simulink model "Coupled_Model_crosslinked_intext"  (R2016a)
settings: Solver=FixedStepDiscrete  StartTime=0  StopTime=1000  FixedStep=1  RelTol=1e-3
undefined symbols (not defined in the file or in its folder): DiscIntNeverNeededParam
libraries: simulink_extras x32
(part 3 of 3)

== matlab function Coupled_Model_crosslinked_intext/kMtcontrol/kMtcontrol2/Spring Function ==
  data: popped output; Lspr input; F output; thresh input; K1 input
function [popped, F] = fcn(Lspr,thresh,K1)
%#eml

rest=0.2e-6;
popLength=0.45e-6;
springLength=0.8e-6;


K2=K1*springLength/(springLength+popLength);

popped=false;


if Lspr < thresh
    F=K1*(Lspr-rest);
    popped=false;

elseif Lspr >= thresh
    F=K2*(Lspr-rest-popLength);
    popped=true;
    
else
    F=0;
end

end

== matlab function Coupled_Model_crosslinked_intext/kMtcontrol/kMtcontrol2/Spring Function  ==
  data: popped output; Lspr input; F output; thresh input; K1 input
function [popped, F] = fcn(Lspr,thresh,K1)
%#eml

rest=0.2e-6;
popLength=0.45e-6;
springLength=0.8e-6;


K2=K1*springLength/(springLength+popLength);

popped=false;


if Lspr < thresh
    F=K1*(Lspr-rest);
    popped=false;

elseif Lspr >= thresh
    F=K2*(Lspr-rest-popLength);
    popped=true;
    
else
    F=0;
end

end

== matlab function Coupled_Model_crosslinked_intext/kMtcontrol/kMtcontrol2/kMt  Dynamics/kMtState/Left Catastophe Function ==
  data: u input; y output
function y = fcn(u)
%#eml
if u < 8e-7
y = -.65*((u*10^6)-0.75).^2+(23/60);
else 
    y=0.389;
end
y=abs(y);

== matlab function Coupled_Model_crosslinked_intext/kMtcontrol/kMtcontrol2/kMt  Dynamics/kMtState/Left Rescue Function ==
  data: u input; y output; v input
function y = fcn(u,v)
%#eml
if v<=0.05e-6
    y=1;
else
    y=-9.5e9*(u)+0.21;
end
y=abs(y);

== matlab function Coupled_Model_crosslinked_intext/kMtcontrol/kMtcontrol2/kMt  Dynamics/kMtState/Right Catastophe Function ==
  data: u input; y output
function y = fcn(u)
%#eml
if u < 8e-7
y = -.65*((u*10^6)-0.75).^2+(23/60);
else 
    y=.389;
end
y=abs(y);

== matlab function Coupled_Model_crosslinked_intext/kMtcontrol/kMtcontrol2/kMt  Dynamics/kMtState/Right Rescue Function ==
  data: u input; y output; v input
function y = fcn(u,v)
%#eml
if v<=0.05e-6
    y=1;
else
    y=-9.5e9*(u)+0.21;
end
y=abs(y);

== matlab function Coupled_Model_crosslinked_intext/kMtcontrol/kMtcontrol2/kMt Dynamics/kMtState/Left Catastophe Function ==
  data: u input; y output
function y = fcn(u)
%#eml
if u < 8e-7
y = -.65*((u*10^6)-0.75).^2+(23/60);
else 
    y=0.389;
end
y=abs(y);

== matlab function Coupled_Model_crosslinked_intext/kMtcontrol/kMtcontrol2/kMt Dynamics/kMtState/Left Rescue Function ==
  data: u input; y output; v input
function y = fcn(u,v)
%#eml
if v<=0.05e-6
    y=1;
else
    y=-9.5e9*(u)+0.21;
end
y=abs(y);

== matlab function Coupled_Model_crosslinked_intext/kMtcontrol/kMtcontrol2/kMt Dynamics/kMtState/Right Catastophe Function ==
  data: u input; y output
function y = fcn(u)
%#eml
if u < 8e-7
y = -.65*((u*10^6)-0.75).^2+(23/60);
else 
    y=.389;
end
y=abs(y);

== matlab function Coupled_Model_crosslinked_intext/kMtcontrol/kMtcontrol2/kMt Dynamics/kMtState/Right Rescue Function ==
  data: u input; y output; v input
function y = fcn(u,v)
%#eml
if v<=0.05e-6
    y=1;
else
    y=-9.5e9*(u)+0.21;
end
y=abs(y);

== matlab function Coupled_Model_crosslinked_intext/kMtcontrol/kMtcontrol2/kMt Dynamics /kMtState/Left Catastophe Function ==
  data: u input; y output
function y = fcn(u)
%#eml
if u < 8e-7
y = -.65*((u*10^6)-0.75).^2+(23/60);
else 
    y=0.389;
end
y=abs(y);

== matlab function Coupled_Model_crosslinked_intext/kMtcontrol/kMtcontrol2/kMt Dynamics /kMtState/Left Rescue Function ==
  data: u input; y output; v input
function y = fcn(u,v)
%#eml
if v<=0.05e-6
    y=1;
else
    y=-9.5e9*(u)+0.21;
end
y=abs(y);

== matlab function Coupled_Model_crosslinked_intext/kMtcontrol/kMtcontrol2/kMt Dynamics /kMtState/Right Catastophe Function ==
  data: u input; y output
function y = fcn(u)
%#eml
if u < 8e-7
y = -.65*((u*10^6)-0.75).^2+(23/60);
else 
    y=.389;
end
y=abs(y);

== matlab function Coupled_Model_crosslinked_intext/kMtcontrol/kMtcontrol2/kMt Dynamics /kMtState/Right Rescue Function ==
  data: u input; y output; v input
function y = fcn(u,v)
%#eml
if v<=0.05e-6
    y=1;
else
    y=-9.5e9*(u)+0.21;
end
y=abs(y);

== matlab function Coupled_Model_crosslinked_intext/kMtcontrol/kMtcontrol2/kMt Dynamics  /kMtState/Left Catastophe Function ==
  data: u input; y output
function y = fcn(u)
%#eml
if u < 8e-7
y = -.65*((u*10^6)-0.75).^2+(23/60);
else 
    y=0.389;
end
y=abs(y);

== matlab function Coupled_Model_crosslinked_intext/kMtcontrol/kMtcontrol2/kMt Dynamics  /kMtState/Left Rescue Function ==
  data: u input; y output; v input
function y = fcn(u,v)
%#eml
if v<=0.05e-6
    y=1;
else
    y=-9.5e9*(u)+0.21;
end
y=abs(y);

== matlab function Coupled_Model_crosslinked_intext/kMtcontrol/kMtcontrol2/kMt Dynamics  /kMtState/Right Catastophe Function ==
  data: u input; y output
function y = fcn(u)
%#eml
if u < 8e-7
y = -.65*((u*10^6)-0.75).^2+(23/60);
else 
    y=.389;
end
y=abs(y);

== matlab function Coupled_Model_crosslinked_intext/kMtcontrol/kMtcontrol2/kMt Dynamics  /kMtState/Right Rescue Function ==
  data: u input; y output; v input
function y = fcn(u,v)
%#eml
if v<=0.05e-6
    y=1;
else
    y=-9.5e9*(u)+0.21;
end
y=abs(y);

== matlab function Coupled_Model_crosslinked_intext/kMtcontrol/kMtcontrol3/ Spring Function ==
  data: popped output; Lspr input; F output; thresh input; K1 input
function [popped, F] = fcn(Lspr,thresh,K1)
%#eml

rest=0.2e-6;
popLength=0.45e-6;
springLength=0.8e-6;


K2=K1*springLength/(springLength+popLength);

popped=false;


if Lspr < thresh
    F=K1*(Lspr-rest);
    popped=false;

elseif Lspr >= thresh
    F=K2*(Lspr-rest-popLength);
    popped=true;
    
else
    F=0;
end

end

== matlab function Coupled_Model_crosslinked_intext/kMtcontrol/kMtcontrol3/ Spring Function  ==
  data: popped output; Lspr input; F output; thresh input; K1 input
function [popped, F] = fcn(Lspr,thresh,K1)
%#eml

rest=0.2e-6;
popLength=0.45e-6;
springLength=0.8e-6;


K2=K1*springLength/(springLength+popLength);

popped=false;


if Lspr < thresh
    F=K1*(Lspr-rest);
    popped=false;

elseif Lspr >= thresh
    F=K2*(Lspr-rest-popLength);
    popped=true;
    
else
    F=0;
end

end

== matlab function Coupled_Model_crosslinked_intext/kMtcontrol/kMtcontrol3/Spring Function ==
  data: popped output; Lspr input; F output; thresh input; K1 input
function [popped, F] = fcn(Lspr,thresh,K1)
%#eml

rest=0.2e-6;
popLength=0.45e-6;
springLength=0.8e-6;


K2=K1*springLength/(springLength+popLength);

popped=false;


if Lspr < thresh
    F=K1*(Lspr-rest);
    popped=false;

elseif Lspr >= thresh
    F=K2*(Lspr-rest-popLength);
    popped=true;
    
else
    F=0;
end

end

== matlab function Coupled_Model_crosslinked_intext/kMtcontrol/kMtcontrol3/Spring Function  ==
  data: popped output; Lspr input; F output; thresh input; K1 input
function [popped, F] = fcn(Lspr,thresh,K1)
%#eml

rest=0.2e-6;
popLength=0.45e-6;
springLength=0.8e-6;


K2=K1*springLength/(springLength+popLength);

popped=false;


if Lspr < thresh
    F=K1*(Lspr-rest);
    popped=false;

elseif Lspr >= thresh
    F=K2*(Lspr-rest-popLength);
    popped=true;
    
else
    F=0;
end

end

== matlab function Coupled_Model_crosslinked_intext/kMtcontrol/kMtcontrol3/kMt  Dynamics/kMtState/Left Catastophe Function ==
  data: u input; y output
function y = fcn(u)
%#eml
if u < 8e-7
y = -.65*((u*10^6)-0.75).^2+(23/60);
else 
    y=0.389;
end
y=abs(y);

== matlab function Coupled_Model_crosslinked_intext/kMtcontrol/kMtcontrol3/kMt  Dynamics/kMtState/Left Rescue Function ==
  data: u input; y output; v input
function y = fcn(u,v)
%#eml
if v<=0.05e-6
    y=1;
else
    y=-9.5e9*(u)+0.21;
end
y=abs(y);

== matlab function Coupled_Model_crosslinked_intext/kMtcontrol/kMtcontrol3/kMt  Dynamics/kMtState/Right Catastophe Function ==
  data: u input; y output
function y = fcn(u)
%#eml
if u < 8e-7
y = -.65*((u*10^6)-0.75).^2+(23/60);
else 
    y=.389;
end
y=abs(y);

== matlab function Coupled_Model_crosslinked_intext/kMtcontrol/kMtcontrol3/kMt  Dynamics/kMtState/Right Rescue Function ==
  data: u input; y output; v input
function y = fcn(u,v)
%#eml
if v<=0.05e-6
    y=1;
else
    y=-9.5e9*(u)+0.21;
end
y=abs(y);

== matlab function Coupled_Model_crosslinked_intext/kMtcontrol/kMtcontrol3/kMt Dynamics/kMtState/Left Catastophe Function ==
  data: u input; y output
function y = fcn(u)
%#eml
if u < 8e-7
y = -.65*((u*10^6)-0.75).^2+(23/60);
else 
    y=0.389;
end
y=abs(y);

== matlab function Coupled_Model_crosslinked_intext/kMtcontrol/kMtcontrol3/kMt Dynamics/kMtState/Left Rescue Function ==
  data: u input; y output; v input
function y = fcn(u,v)
%#eml
if v<=0.05e-6
    y=1;
else
    y=-9.5e9*(u)+0.21;
end
y=abs(y);

== matlab function Coupled_Model_crosslinked_intext/kMtcontrol/kMtcontrol3/kMt Dynamics/kMtState/Right Catastophe Function ==
  data: u input; y output
function y = fcn(u)
%#eml
if u < 8e-7
y = -.65*((u*10^6)-0.75).^2+(23/60);
else 
    y=.389;
end
y=abs(y);

== matlab function Coupled_Model_crosslinked_intext/kMtcontrol/kMtcontrol3/kMt Dynamics/kMtState/Right Rescue Function ==
  data: u input; y output; v input
function y = fcn(u,v)
%#eml
if v<=0.05e-6
    y=1;
else
    y=-9.5e9*(u)+0.21;
end
y=abs(y);

== matlab function Coupled_Model_crosslinked_intext/kMtcontrol/kMtcontrol3/kMt Dynamics /kMtState/Left Catastophe Function ==
  data: u input; y output
function y = fcn(u)
%#eml
if u < 8e-7
y = -.65*((u*10^6)-0.75).^2+(23/60);
else 
    y=0.389;
end
y=abs(y);

== matlab function Coupled_Model_crosslinked_intext/kMtcontrol/kMtcontrol3/kMt Dynamics /kMtState/Left Rescue Function ==
  data: u input; y output; v input
function y = fcn(u,v)
%#eml
if v<=0.05e-6
    y=1;
else
    y=-9.5e9*(u)+0.21;
end
y=abs(y);

== matlab function Coupled_Model_crosslinked_intext/kMtcontrol/kMtcontrol3/kMt Dynamics /kMtState/Right Catastophe Function ==
  data: u input; y output
function y = fcn(u)
%#eml
if u < 8e-7
y = -.65*((u*10^6)-0.75).^2+(23/60);
else 
    y=.389;
end
y=abs(y);

== matlab function Coupled_Model_crosslinked_intext/kMtcontrol/kMtcontrol3/kMt Dynamics /kMtState/Right Rescue Function ==
  data: u input; y output; v input
function y = fcn(u,v)
%#eml
if v<=0.05e-6
    y=1;
else
    y=-9.5e9*(u)+0.21;
end
y=abs(y);

== matlab function Coupled_Model_crosslinked_intext/kMtcontrol/kMtcontrol3/kMt Dynamics  /kMtState/Left Catastophe Function ==
  data: u input; y output
function y = fcn(u)
%#eml
if u < 8e-7
y = -.65*((u*10^6)-0.75).^2+(23/60);
else 
    y=0.389;
end
y=abs(y);

== matlab function Coupled_Model_crosslinked_intext/kMtcontrol/kMtcontrol3/kMt Dynamics  /kMtState/Left Rescue Function ==
  data: u input; y output; v input
function y = fcn(u,v)
%#eml
if v<=0.05e-6
    y=1;
else
    y=-9.5e9*(u)+0.21;
end
y=abs(y);

== matlab function Coupled_Model_crosslinked_intext/kMtcontrol/kMtcontrol3/kMt Dynamics  /kMtState/Right Catastophe Function ==
  data: u input; y output
function y = fcn(u)
%#eml
if u < 8e-7
y = -.65*((u*10^6)-0.75).^2+(23/60);
else 
    y=.389;
end
y=abs(y);

== matlab function Coupled_Model_crosslinked_intext/kMtcontrol/kMtcontrol3/kMt Dynamics  /kMtState/Right Rescue Function ==
  data: u input; y output; v input
function y = fcn(u,v)
%#eml
if v<=0.05e-6
    y=1;
else
    y=-9.5e9*(u)+0.21;
end
y=abs(y);

== matlab function Coupled_Model_crosslinked_intext/kMtcontrol/kMtcontrol/kMt Dynamics /kMtState/Left Catastophe Function ==
  data: u input; y output
function y = fcn(u)
%#eml
if u < 8e-7
y = -.65*((u*10^6)-0.75).^2+(23/60);
else 
    y=0.389;
end
y=abs(y);

== matlab function Coupled_Model_crosslinked_intext/kMtcontrol/kMtcontrol/kMt Dynamics /kMtState/Left Rescue Function ==
  data: u input; y output; v input
function y = fcn(u,v)
%#eml
if v<=0.05e-6
    y=1;
else
    y=-9.5e9*(u)+0.21;
end
y=abs(y);

== matlab function Coupled_Model_crosslinked_intext/kMtcontrol/kMtcontrol/kMt Dynamics /kMtState/Right Catastophe Function ==
  data: u input; y output
function y = fcn(u)
%#eml
if u < 8e-7
y = -.65*((u*10^6)-0.75).^2+(23/60);
else 
    y=.389;
end
y=abs(y);

== matlab function Coupled_Model_crosslinked_intext/kMtcontrol/kMtcontrol/kMt Dynamics /kMtState/Right Rescue Function ==
  data: u input; y output; v input
function y = fcn(u,v)
%#eml
if v<=0.05e-6
    y=1;
else
    y=-9.5e9*(u)+0.21;
end
y=abs(y);

== matlab function Coupled_Model_crosslinked_intext/kMtcontrol/kMtcontrol/kMt  Dynamics/kMtState/Left Catastophe Function ==
  data: u input; y output
function y = fcn(u)
%#eml
if u < 8e-7
y = -.65*((u*10^6)-0.75).^2+(23/60);
else 
    y=0.389;
end
y=abs(y);

== matlab function Coupled_Model_crosslinked_intext/kMtcontrol/kMtcontrol/kMt  Dynamics/kMtState/Left Rescue Function ==
  data: u input; y output; v input
function y = fcn(u,v)
%#eml
if v<=0.05e-6
    y=1;
else
    y=-9.5e9*(u)+0.21;
end
y=abs(y);

== matlab function Coupled_Model_crosslinked_intext/kMtcontrol/kMtcontrol/kMt  Dynamics/kMtState/Right Catastophe Function ==
  data: u input; y output
function y = fcn(u)
%#eml
if u < 8e-7
y = -.65*((u*10^6)-0.75).^2+(23/60);
else 
    y=.389;
end
y=abs(y);

== matlab function Coupled_Model_crosslinked_intext/kMtcontrol/kMtcontrol/kMt  Dynamics/kMtState/Right Rescue Function ==
  data: u input; y output; v input
function y = fcn(u,v)
%#eml
if v<=0.05e-6
    y=1;
else
    y=-9.5e9*(u)+0.21;
end
y=abs(y);

== matlab function Coupled_Model_crosslinked_intext/kMtcontrol/kMtcontrol/kMt Dynamics  /kMtState/Left Catastophe Function ==
  data: u input; y output
function y = fcn(u)
%#eml
if u < 8e-7
y = -.65*((u*10^6)-0.75).^2+(23/60);
else 
    y=0.389;
end
y=abs(y);

== matlab function Coupled_Model_crosslinked_intext/kMtcontrol/kMtcontrol/kMt Dynamics  /kMtState/Left Rescue Function ==
  data: u input; y output; v input
function y = fcn(u,v)
%#eml
if v<=0.05e-6
    y=1;
else
    y=-9.5e9*(u)+0.21;
end
y=abs(y);

== matlab function Coupled_Model_crosslinked_intext/kMtcontrol/kMtcontrol/kMt Dynamics  /kMtState/Right Catastophe Function ==
  data: u input; y output
function y = fcn(u)
%#eml
if u < 8e-7
y = -.65*((u*10^6)-0.75).^2+(23/60);
else 
    y=.389;
end
y=abs(y);

== matlab function Coupled_Model_crosslinked_intext/kMtcontrol/kMtcontrol/kMt Dynamics  /kMtState/Right Rescue Function ==
  data: u input; y output; v input
function y = fcn(u,v)
%#eml
if v<=0.05e-6
    y=1;
else
    y=-9.5e9*(u)+0.21;
end
y=abs(y);

== matlab function Coupled_Model_crosslinked_intext/Polcontrol/Embedded MATLAB Function2 ==
  data: Fnet input; Vip output
function Vip=fcn(Fnet)
%#eml

% if Fnet < 6e-12
    Vip=(50e-9/6e-12)*Fnet;
% else
%     Vip=50e-9;
% end

== matlab function Coupled_Model_crosslinked_intext/Polcontrol/Embedded MATLAB Function3 ==
  data: Fnet input; y output; Nmotors input
function y = fcn(Fnet,Nmotors)
%#eml
if Nmotors == 0
    y = 0;
else
    y = Fnet/Nmotors;
end

== matlab function Coupled_Model_crosslinked_intext/kMtcontrol/kMtcontrol/Spring Function ==
  data: popped output; Lspr input; F output; thresh input; K1 input
function [popped, F] = fcn(Lspr,thresh,K1)
%#eml

rest=0.2e-6;
popLength=0.45e-6;
springLength=0.8e-6;


K2=K1*springLength/(springLength+popLength);

popped=false;


if Lspr < thresh
    F=K1*(Lspr-rest);
    popped=false;

elseif Lspr >= thresh
    F=K2*(Lspr-rest-popLength);
    popped=true;
    
else
    F=0;
end

end

== matlab function Coupled_Model_crosslinked_intext/kMtcontrol/kMtcontrol/Spring Function  ==
  data: popped output; Lspr input; F output; thresh input; K1 input
function [popped, F] = fcn(Lspr,thresh,K1)
%#eml

rest=0.2e-6;
popLength=0.45e-6;
springLength=0.8e-6;


K2=K1*springLength/(springLength+popLength);

popped=false;


if Lspr < thresh
    F=K1*(Lspr-rest);
    popped=false;

elseif Lspr >= thresh
    F=K2*(Lspr-rest-popLength);
    popped=true;
    
else
    F=0;
end

end

== matlab function Coupled_Model_crosslinked_intext/kMtcontrol/kMtcontrol/ Spring Function  ==
  data: popped output; Lspr input; F output; thresh input; K1 input
function [popped, F] = fcn(Lspr,thresh,K1)
%#eml

rest=0.2e-6;
popLength=0.45e-6;
springLength=0.8e-6;


K2=K1*springLength/(springLength+popLength);

popped=false;


if Lspr < thresh
    F=K1*(Lspr-rest);
    popped=false;

elseif Lspr >= thresh
    F=K2*(Lspr-rest-popLength);
    popped=true;
    
else
    F=0;
end

end

== matlab function Coupled_Model_crosslinked_intext/kMtcontrol/kMtcontrol/ Spring Function ==
  data: popped output; Lspr input; F output; thresh input; K1 input
function [popped, F] = fcn(Lspr,thresh,K1)
%#eml

rest=0.2e-6;
popLength=0.45e-6;
springLength=0.8e-6;


K2=K1*springLength/(springLength+popLength);

popped=false;


if Lspr < thresh
    F=K1*(Lspr-rest);
    popped=false;

elseif Lspr >= thresh
    F=K2*(Lspr-rest-popLength);
    popped=true;
    
else
    F=0;
end

end

== matlab function Coupled_Model_crosslinked_intext/kMtcontrol/kMtcontrol/kMt Dynamics/kMtState/Left Catastophe Function ==
  data: u input; y output
function y = fcn(u)
%#eml
if u < 8e-7
y = -.65*((u*10^6)-0.75).^2+(23/60);
else 
    y=0.389;
end
y=abs(y);

== matlab function Coupled_Model_crosslinked_intext/kMtcontrol/kMtcontrol/kMt Dynamics/kMtState/Left Rescue Function ==
  data: u input; y output; v input
function y = fcn(u,v)
%#eml
if v<=0.05e-6
    y=1;
else
    y=-9.5e9*(u)+0.21;
end
y=abs(y);

== matlab function Coupled_Model_crosslinked_intext/kMtcontrol/kMtcontrol/kMt Dynamics/kMtState/Right Catastophe Function ==
  data: u input; y output
function y = fcn(u)
%#eml
if u < 8e-7
y = -.65*((u*10^6)-0.75).^2+(23/60);
else 
    y=.389;
end
y=abs(y);

== matlab function Coupled_Model_crosslinked_intext/kMtcontrol/kMtcontrol/kMt Dynamics/kMtState/Right Rescue Function ==
  data: u input; y output; v input
function y = fcn(u,v)
%#eml
if v<=0.05e-6
    y=1;
else
    y=-9.5e9*(u)+0.21;
end
y=abs(y);
